simulink model "PID_4opamp_blocks"  (R2019b)
settings: Solver=VariableStepAuto  StartTime=0.0  StopTime=15  RelTol=1e-3
settings Model: Creator=robom  LastModifiedBy=robom
settings DataIOCC: SaveOutput=off  ReturnWorkspaceOutputs=off
settings DebuggingCC: AlgebraicLoopMsg=none
settings SFSimCC: CustomCodeUndefinedFunction=UseInterfaceOnly

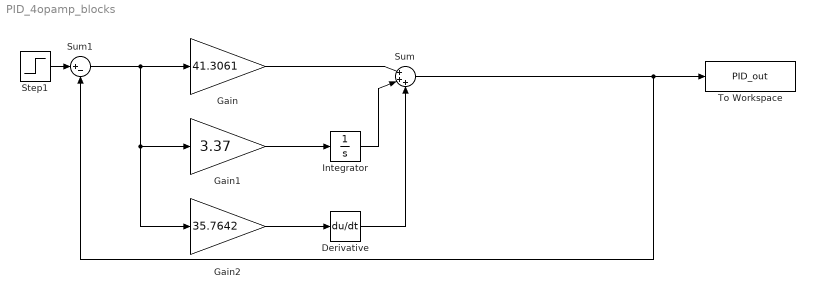
== system PID_4opamp_blocks ==
  Derivative : Derivative
  Gain : Gain  Gain=41.3061
  Gain1 : Gain  Gain=3.37
  Gain2 : Gain  Gain=35.7642
  Integrator : Integrator
  Step1 : Step  Time=0  SampleTime=0
  Sum : Sum  Inputs=|+++
  Sum1 : Sum  Inputs=|+-
  To Workspace : ToWorkspace  VariableName=PID_out  SampleTime=-1
      settings: Save2DSignal=2-D array (concatenate along first dimension)
  wires:
  Step1/1 -> Sum1/1
  Sum/1 -> To Workspace/1, Sum1/2
  Gain2/1 -> Derivative/1
  Gain1/1 -> Integrator/1
  Derivative/1 -> Sum/3
  Integrator/1 -> Sum/2
  Gain/1 -> Sum/1
  Sum1/1 -> Gain2/1, Gain1/1, Gain/1
